simulink model "BACKUP"  (R2023b)
settings: Solver=VariableStepAuto  StartTime=0.0  StopTime=10.0  RelTol=1e-3
values from neighbouring files (symbols this model uses):
  C_PM = 1.758e-3    (= 0.001758)    [HVDCMMCInterconnectionParam.m]
  Carm = C_PM/Nb_PM    (= 4.88333333333e-05)    [HVDCMMCInterconnectionParam.m]
  Cfilter = 1/(Larm*wc2)    (= 4.78421193241e-05)    [HVDCMMCInterconnectionParam.m]
  Cg = 50e-9    (= 5e-08)    [HVDCMMCInterconnectionParam.m]
  Dd11 = Dd(1:nsw,1:nsw);        if(isempty(Dd11)) Dd11 = zeros(3,3); end    [DSS.m]    (also in DSS_test.m)
  Dd12 = Dd(1:nsw,nsw+1:end);    if(isempty(Dd12)) Dd12 = zeros(3,3); end    [DSS.m]    (also in DSS_test.m)
  Fnom = 50    [HVDCMMCInterconnectionParam.m]
  HRM = 2    [HVDCMMCInterconnectionParam.m]
  Ib_ac = (2/3)*Pnom/Vb_ac    [HVDCMMCInterconnectionParam.m]
  Ki_Ireg = 6    [HVDCMMCInterconnectionParam.m]
  Ki_Preg = 1.0    (= 1)    [HVDCMMCInterconnectionParam.m]
  Ki_Qreg = 1.0    (= 1)    [HVDCMMCInterconnectionParam.m]
  Ki_VDCreg = 100    [HVDCMMCInterconnectionParam.m]
  Kp_Ireg = 0.6    [HVDCMMCInterconnectionParam.m]
  Kp_Preg = 0.5/3    (= 0.166666666667)    [HVDCMMCInterconnectionParam.m]
  Kp_Qreg = 0.5/3    (= 0.166666666667)    [HVDCMMCInterconnectionParam.m]
  Kp_VDCreg = 4    [HVDCMMCInterconnectionParam.m]
  L_cable = 15e-3    (= 0.015)    [HVDCMMCInterconnectionParam.m]
  Larm = Larm_pu*(Zb_ac/(2*pi*Fnom))    [HVDCMMCInterconnectionParam.m]
  Lff = Larm_pu/2    (= 0.075)    [HVDCMMCInterconnectionParam.m]
  Limits_Ireg = [ 2.0  -2.0]    [HVDCMMCInterconnectionParam.m]
  Limits_Preg = [ 1.2, 0.8 ]    [HVDCMMCInterconnectionParam.m]
  Limits_Qreg = [ 0.25, -0.25 ]    [HVDCMMCInterconnectionParam.m]
  Limits_VDCreg = [ 2.0  -2.0]    [HVDCMMCInterconnectionParam.m]
  Lxfo = 0.12    [HVDCMMCInterconnectionParam.m]
  Nb_PM = 36    [HVDCMMCInterconnectionParam.m]
  Pnom = 1000e6    (= 1000000000)    [HVDCMMCInterconnectionParam.m]
  R_cable = 0.5    [HVDCMMCInterconnectionParam.m]
  R_startup = 400    [HVDCMMCInterconnectionParam.m]
  Rarm = Rarm_pu*Zb_ac    [HVDCMMCInterconnectionParam.m]
  Rff = Rarm_pu/2    (= 0.00075)    [HVDCMMCInterconnectionParam.m]
  Rfilter = 1/(Cfilter*w)*30    (= 1996.002)    [HVDCMMCInterconnectionParam.m]
  Rg = 100    [HVDCMMCInterconnectionParam.m]
  Rxfo = 0.003    [HVDCMMCInterconnectionParam.m]
  Ts = Ts_Control    (= 4e-05)    [HVDCMMCInterconnectionParam.m]
  Ts_Control = 40e-6    (= 4e-05)    [HVDCMMCInterconnectionParam.m]
  Ts_Power = 20e-6    (= 2e-05)    [HVDCMMCInterconnectionParam.m]
  Vb_ac = sqrt(2/3)*Vnom_sec    [HVDCMMCInterconnectionParam.m]
  Vc0_PM = 0    [HVDCMMCInterconnectionParam.m]
  Vnom_dc = 640e3    (= 640000)    [HVDCMMCInterconnectionParam.m]
  Vnom_prim = 400e3    (= 400000)    [HVDCMMCInterconnectionParam.m]
  Vnom_sec = 333e3    (= 333000)    [HVDCMMCInterconnectionParam.m]
  w = 2*pi*Fnom    (= 314.159265359)    [HVDCMMCInterconnectionParam.m]
  Zb_ac = Vb_ac/Ib_ac    [HVDCMMCInterconnectionParam.m]
undefined symbols (not defined in the file or in its folder): Ad1, Bd1, Cd1, DiscIntNeverNeededParam, gcbh, HrmOrd, Pcc, sps_AC, sps_ACDC, sps_rtmsupport, SYS, Ts_EMT
libraries: spsSeriesRLCBranchLib x22, simulink x20, spsCurrentMeasurementLib x13, spsControlledVoltageSourceLib x12, DQN_Lib x9, spsdq0toabcLib x3, powerlib_extras x3, spsGroundLib x3, spsBreakerLib x3, spsParallelRLCBranchLib x3, eeGeneralControl x2, dspspect3 x2
(part 1 of 5)
settings Model: Creator=rober  LastModifiedBy=rober

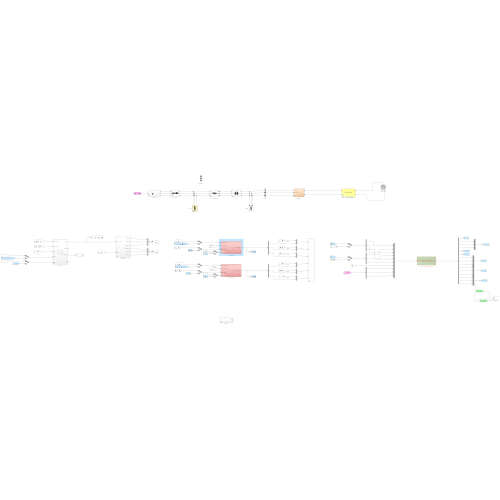
[thumbnail: Simulink's stored preview of the top-level diagram]
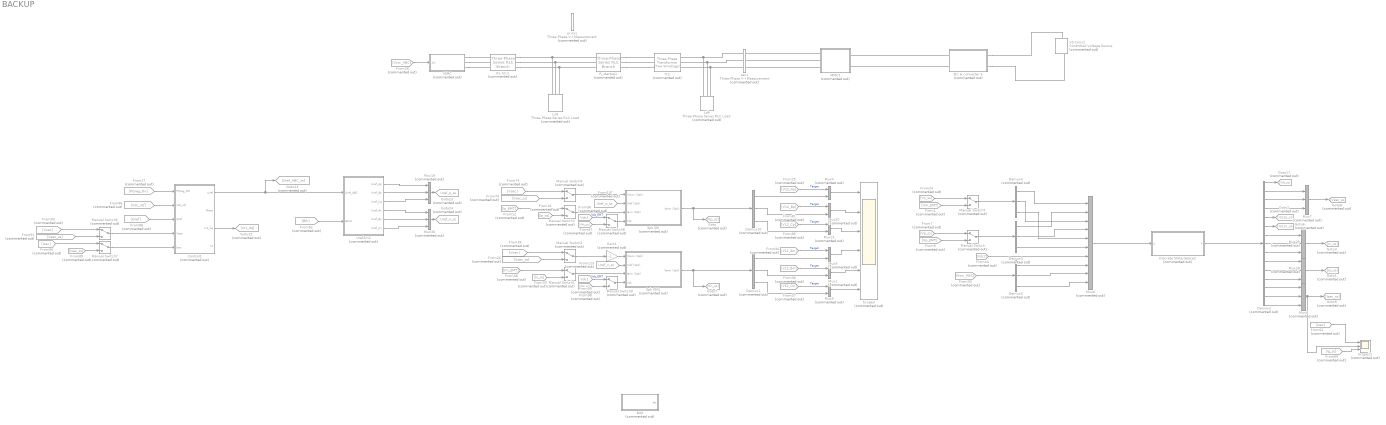
== system BACKUP ==
  3ph SM : Subsystem  Commented=on
  3ph SM1 : Subsystem  Commented=on
  BAK : Subsystem  Commented=on
  Control1 : Subsystem  Commented=on
  DC & converter 3 : Subsystem  Commented=on
      mask Display: disp('DC circuit')
  Demux{1,3..5,10} (5 alike) : Demux  Commented=on  Outputs=3
  Demux2 : Demux  Commented=on  Outputs=numel(sps_ACDC.outputs)
  Discrete State-Space2 : Subsystem  Commented=on  SystemSampleTime=Ts_Power  mask{A=sps_ACDC.A, B=sps_ACDC.B, C=sps_ACDC.C, D=sps_ACDC.D, InitVec=sps_ACDC.x0, dt=Ts_Power, DQSYM=off, N=HRM, Ws=w}
      mask prompts: InitVec "Initial condition:"; dt "Time step (s):"; N "Harmonic number:"; Ws "Angular frequency (1/rad):"
      mask init:
      | % I = eye(size(A,1));
      | % INVR = I/(I-A*dt/2);
      | % Ad1 = INVR*(I+A*dt/2);
      | % Bd1 = INVR*B*dt/2;
      | % Cd1 = C*Ad1;
      | % Dd11 = C*INVR*B*dt/2+D;
      | % Dd12 = C*INVR*B*dt/2;
      | 
      |     I = eye(size(A,1));
      |     INVR = I/(I-A*dt/2);
      |     Ad1 = INVR*(I+A*dt/2);
      |     Bd1 = INVR*B;
      |     Cd1 = C*INVR*dt;
      |     Dd1 = Cd1*B/2 + D;
      | 
      | DQSYM = get_param(gcb,'DQSYM');
      | 
      | comp = 0;
      | 
      | if(strcmp(DQSYM,'on'))
      | 
      | %Calculating the PNZ matrices
      | 
      |     a = -0.5+0.866i;
      |     a2 = -0.5-0.866i;
      |     Sas = [1,a,a2;1,a2,a;1,1,1]/3;
      | 
      |     arows = size(Ad1,1)/3; %signal size
      |     acols = size(Ad1,2)/3; %signal size
      | 
      |     brows = size(Bd1,1)/3; %signal size
      |     bcols = size(Bd1,2)/3; %signal size
      | 
      |     crows = size(Cd1,1)/3; %signal size
      |     ccols = size(Cd1,2)/3; %signal size
      | 
      |     d1rows = size(Dd1,1)/3; %signal size
      |     d1cols = size(Dd1,2)/3; %signal size
      | 
      |     %%%%%%%%%%%%%%%%%%%%%%% Check for inconsistencies  %%%%%%%%%%%%%%%%%%%%%%%
      | 
      |     szMatA = size(A,1);
      |     iL = eye(szMatA);
      |     szMatiL = size(iL,1);
      | 
      |     if(szMatiL ~= szMatA || size(A,1) ~= size(A,2) || size(iL,1) ~= size(iL,2))
      |         error('[Int_DQN_Mat/swFeedback] check matrix A size!');
      |     end
      | 
      |     if(arows ~= brows || acols ~= ccols || crows ~= d1rows || bcols ~= d1cols)
      |         error('[Int_DQN_Mat/Initialize] the sizes of the state-space matrices!');
      |     end
      | 
      |     %%%%%%%%%%%%%%%%%%%%%%%%%%%%%%%%%%%%%%%%%%%%%%%%%%%%%%%%%%%%%%%
      | 
      | 
      |     %%%%%%%%%%%%%%%%%%%%%%% A --> Bpnz %%%%%%%%%%%%%%%%%%%%%%%
      |     Adc = complex(zeros(3*arows,3*acols));
      | 
      |     for i = 1 : arows
      |         for j = 1 : acols
      |             Adc((1:3) + (i-1)*3,(1:3) + (j-1)*3) = Sas*Ad1((1:3) + (i-1)*3,(1:3) + (j-1)*3)/Sas;
      |             %Adc((1:3) + (i-1)*3,(1:3) + (j-1)*3) = diag(diag(real(Adc((1:3) + (i-1)*3,(1:3) + (j-1)*3))));
      |             %Adc((1:3) + (i-1)*3,(1:3) + (j-1)*3) = diag(diag((Adc((1:3) + (i-1)*3,(1:3) + (j-1)*3))));
      | 
      |         end
      |     end
      |     %%%%%%%%%%%%%%%%%%%%%%%%%%%%%%%%%%%%%%%%%%%%%%%%%%%%%%%%%%%%%%%
      | 
      |     %%%%%%%%%%%%%%%%%%%%%%% B --> Bpnz %%%%%%%%%%%%%%%%%%%%%%%
      | 
      |     Bdc = complex(zeros(3*brows,3*bcols));
      | 
      |     for i = 1 : brows
      |         for j = 1 : bcols
      |             Bdc((1:3) + (i-1)*3,(1:3) + (j-1)*3) = Sas*Bd1((1:3) + (i-1)*3,(1:3) + (j-1)*3)/Sas;
      |             %Bdc((1:3) + (i-1)*3,(1:3) + (j-1)*3) = diag(diag(real(Bdc((1:3) + (i-1)*3,(1:3) + (j-1)*3))));
      |             %Bdc((1:3) + (i-1)*3,(1:3) + (j-1)*3) = diag(diag((Bdc((1:3) + (i-1)*3,(1:3) + (j-1)*3))));
      | 
      |         end
      |     end
      |     %%%%%%%%%%%%%%%%%%%%%%%%%%%%%%%%%%%%%%%%%%%%%%%%%%%%%%%%%%%%%%%
      | 
      |     %%%%%%%%%%%%%%%%%%%%%%% C --> Cpnz %%%%%%%%%%%%%%%%%%%%%%%
      | 
      |     Cdc = complex(zeros(3*crows,3*ccols));
      | 
      |     for i = 1 : crows
      |         for j = 1 : ccols
      |             Cdc((1:3) + (i-1)*3,(1:3) + (j-1)*3) = Sas*Cd1((1:3) + (i-1)*3,(1:3) + (j-1)*3)/Sas;
      |             %Cdc((1:3) + (i-1)*3,(1:3) + (j-1)*3) = diag(diag(real(Cdc((1:3) + (i-1)*3,(1:3) + (j-1)*3))));
      |             %Cdc((1:3) + (i-1)*3,(1:3) + (j-1)*3) = diag(diag((Cdc((1:3) + (i-1)*3,(1:3) + (j-1)*3))));
      |         end
      |     end
      |     %%%%%%%%%%%%%%%%%%%%%%%%%%%%%%%%%%%%%%%%%%%%%%%%%%%%%%%%%%%%%%%
      | 
      |     
      |     %%%%%%%%%%%%%%%%%%%%%%% D1 --> Cpnz %%%%%%%%%%%%%%%%%%%%%%%
      | 
      |     Ddc = complex(zeros(3*d1rows,3*d1cols));
      | 
      |     for i = 1 : d1rows
      |         for j = 1 : d1cols
      |             Ddc((1:3) + (i-1)*3,(1:3) + (j-1)*3) = Sas*Dd1((1:3) + (i-1)*3,(1:3) + (j-1)*3)/Sas;
      |             %Ddc1((1:3) + (i-1)*3,(1:3) + (j-1)*3) = diag(diag(real(Ddc1((1:3) + (i-1)*3,(1:3) + (j-1)*3))));
      |             %Ddc((1:3) + (i-1)*3,(1:3) + (j-1)*3) = diag(diag((Ddc((1:3) + (i-1)*3,(1:3) + (j-1)*3))));
      |         end
      |     end
      |     %%%%%%%%%%%%%%%%%%%%%%%%%%%%%%%%%%%%%%%%%%%%%%%%%%%%%%%%%%%%%%%
      | 
      |     Adc(abs(Adc)<2*eps) = 0;
      |     Bdc(abs(Bdc)<2*eps) = 0;
      |     Cdc(abs(Cdc)<2*eps) = 0;
      |     Ddc(abs(Ddc)<2*eps) = 0;
      | 
      |     InitVec_c = complex(zeros(brows*3,N+1));
      | 
      | 
      |     if(~isempty(InitVec))
      |         if(mod(numel(InitVec),3)~=0) 
      |             warning('[SS_DQNc_Mat] InitVec with wrong size --> needs to be a multiple of 3!'); 
      | 
      |         else
      |             for k = 1 : numel(InitVec)/3
      |                 InitVec_c((k-1)*3+1:(k-1)*3+3,1) = Sas*InitVec((k-1)*3+1:(k-1)*3+3)*exp(+1i*Ws*dt);
      |             end
      |         end
      |     end
      | 
      |     InitVec = InitVec_c;
      | 
      | 
      |     Ad1 = Adc;
      |     Bd1 = Bdc;
      |     Cd1 = Cdc;
      |     Dd1 = Ddc;
      | 
      |     comp = -1i*Ws*dt;
      | 
      | end
      settings: MinAlgLoopOccurrences=on
      settings: LibrarySourceBlock=|
      | spsSynchronousMachineModel/Discrete robust/State Space Model/Discretize
      | BE or Tustin
      mask Callback DQSYM:
      | EMT = get_param(gcb,'DQSYM');
      | 
      | if(strcmp(EMT,'on'))
      |    set_param(gcb,'MaskVisibilities',{'on','on','on','on','on','on','on','on','on'});
      | else
      |    set_param(gcb,'MaskVisibilities',{'on','on','on','on','on','on','on','off','off'});
      | end
      mask Display: disp(['{\color{red}\bf\fontsize{12}x(t) = Ad*x(t-dt)+Bd*u(t)}',newline,'{\color{gray}\bf\fontsize{12}y(t) = Cd*x(t-dt)+Dd*u(t)}'], 'texmode','on');
  From1 : From  Commented=on  GotoTag=Vm_EMT
  From107 : From  Commented=on  GotoTag=Uref_p_ss  TagVisibility=global
  From113 : From  Commented=on  GotoTag=Uref_n_ss  TagVisibility=global
  From12 : From  Commented=on  GotoTag=Ip_EMT
  From16 : From  Commented=on  GotoTag=Ip_ss
  From24 : From  Commented=on  GotoTag=Vn_ss
  From25 : From  Commented=on  GotoTag=V12_Ap  TagVisibility=global
  From26 : From  Commented=on  GotoTag=Vsec_ss
  From27 : From  Commented=on  GotoTag=PQreg_On  TagVisibility=global
  From28 : From  Commented=on  GotoTag=Vsrc_ABC
  From30 : From  Commented=on  GotoTag=Vsrc_ABC
  From33 : From  Commented=on  GotoTag=In_ss
  From34 : From  Commented=on  GotoTag=V12_Am  TagVisibility=global
  From36 : From  Commented=on  GotoTag=V12_Bm  TagVisibility=global
  From37 : From  Commented=on  GotoTag=V12_Cm  TagVisibility=global
  From39 : From  Commented=on  GotoTag=Vsec  TagVisibility=global
  From44 : From  Commented=on  GotoTag=Vdc2  TagVisibility=global
  From48 : From  Commented=on  GotoTag=Im_EMT
  From62 : From  Commented=on  GotoTag=Isec  TagVisibility=global
  From69 : From  Commented=on  GotoTag=Ig_ss
  From7 : From  Commented=on  GotoTag=Vp_ss
  From73 : From  Commented=on  GotoTag=Vsec_ss
  From74 : From  Commented=on  GotoTag=Vsec  TagVisibility=global
  From81 : From  Commented=on  GotoTag=V12_Bp  TagVisibility=global
  From85 : From  Commented=on  GotoTag=V12_Cp  TagVisibility=global
  From86 : From  Commented=on  GotoTag=Vdc_ref  TagVisibility=global
  From87 : From  Commented=on  GotoTag=Vdc_ss
  From88 : From  Commented=on  GotoTag=Qref  TagVisibility=global
  From89 : From  Commented=on  GotoTag=Isec_ss
  From9 : From  Commented=on  GotoTag=Vp_EMT
  From90 : From  Commented=on  GotoTag=Isec  TagVisibility=global
  From91 : From  Commented=on  GotoTag=Vsec_ss
  From92 : From  Commented=on  GotoTag=Blk  TagVisibility=global
  From93 : From  Commented=on  GotoTag=Vsec  TagVisibility=global
  From96 : From  Commented=on  GotoTag=Vdc1  TagVisibility=global
  From98 : From  Commented=on  GotoTag=Vdc_ss
  From99 : From  Commented=on  GotoTag=Vdc1  TagVisibility=global
  Gain1 : Gain  Commented=on  Gain=-1
  Goto : Goto  Commented=on  GotoTag=Vp_ss
  Goto1 : Goto  Commented=on  GotoTag=Ip_ss
  Goto13 : Goto  Commented=on  GotoTag=Uref_ABC_ss
  Goto15 : Goto  Commented=on  GotoTag=m1_dq
  Goto17 : Goto  Commented=on  GotoTag=Vdc_ss
  Goto2 : Goto  Commented=on  GotoTag=Idc1p_ss
  Goto23 : Goto  Commented=on  GotoTag=Uref_p_ss  TagVisibility=global
  Goto24 : Goto  Commented=on  GotoTag=Uref_n_ss  TagVisibility=global
  Goto3 : Goto  Commented=on  GotoTag=In_ss
  Goto6 : Goto  Commented=on  GotoTag=Idc1n_ss
  Goto7 : Goto  Commented=on  GotoTag=Vn_ss
  Goto8 : Goto  Commented=on  GotoTag=Vsec_ss
  Goto9 : Goto  Commented=on  GotoTag=Isec_ss
  Ld3 : spsThreePhaseSeriesRLCLoadLib/Three-Phase Series RLC Load  Commented=on  LConnTagsString=A|B|C  Configuration=Y (grounded)  NominalVoltage=Vnom_prim  Vabc=[1e3 1e3 1e3]  Vabcp=[1e3 1e3 1e3]  NominalFrequency=Fnom  UnbalancedPower=off  ActivePower=P_Ld1  InductivePower=0  CapacitivePower=0  Pabc=[10e3 9e3 11e3]  QLabc=[100 90 110]  QCabc=[100 90 110]  Pabcp=[10e3 9e3 11e3]  QLabcp=[100 90 110]  QCabcp=[100 90 110]  Measurements=None  LoadType=constant Z
  Ld4 : spsThreePhaseSeriesRLCLoadLib/Three-Phase Series RLC Load  Commented=on  LConnTagsString=A|B|C  Configuration=Y (grounded)  NominalVoltage=Vnom_sec  Vabc=[1e3 1e3 1e3]  Vabcp=[1e3 1e3 1e3]  NominalFrequency=Fnom  UnbalancedPower=off  ActivePower=500e3  InductivePower=0  CapacitivePower=0  Pabc=[10e3 9e3 11e3]  QLabc=[100 90 110]  QCabc=[100 90 110]  Pabcp=[10e3 9e3 11e3]  QLabcp=[100 90 110]  QCabcp=[100 90 110]  Measurements=None  LoadType=constant Z
  MMC1 : Subsystem  Commented=on
  Manual Switch{,1..9} (10 alike) : ManualSwitch  Commented=on
  Mux{1,4..5,9,20..21} (6 alike) : Mux  Commented=on  Inputs=2
  Mux{7..8,19,28..30} (6 alike) : Mux  Commented=on  Inputs=3
  Mux6 : Mux  Commented=on  Inputs=numel(sps_ACDC.inputs)
  RL Src1 : spsThreePhaseSeriesRLCBranchLib/Three-Phase Series RLC Branch  Commented=on  LConnTagsString=A|B|C  RConnTagsString=A|B|C  BranchType=RL  Resistance=0.8929  Inductance=16.58e-3  Capacitance=1e-6  Measurements=None
  R_startup1 : spsThreePhaseSeriesRLCBranchLib/Three-Phase Series RLC Branch  Commented=on  LConnTagsString=A|B|C  RConnTagsString=A|B|C  BranchType=R  Resistance=R_startup/50  Inductance=Vnom_prim^2 / Pcc / (2*pi*Fnom)  Capacitance=1e-6  Measurements=None
  Scope11 : Scope  Commented=on  NumInputPorts=3
  Scope3 : Scope  Commented=on  NumInputPorts=6
  Tr2 : spsThreePhaseTransformerTwoWindingsLib/Three-Phase Transformer (Two Windings)  Commented=on  Winding1Connection=Yg  Winding2Connection=Yg  CoreType=Three single-phase transformers  SetSaturation=off  Hysteresis=off  DataFile='hysteresis'  SetInitialFlux=off  Measurements=None  UNITS=pu  NominalPower=[ Pnom , Fnom ]  Winding1="[ Vnom_prim , Rxfo/2,  Lxfo/2 ]"  Winding2="[ Vnom_sec , Rxfo/2,  Lxfo/2 ]"  Rm=1000  Lm=1000  L0=0.5  Saturation=[ 0,0 ; 0.0024,1.2 ; 1.0,1.52 ]  InitialFluxes=[ 0.8 , -0.8 , 0.7 ]  BreakLoop=off  DiscreteSolver=Trapezoidal iterative  DataType=off  TransfoNumber=1
  Uref2m2 : Subsystem  Commented=on
  VS Conv2 : spsControlledVoltageSourceLib/Controlled Voltage Source  Commented=on  Initialize=on  Source_Type=AC  Amplitude=0  Phase=0  Frequency=0  Measurements=None
  VSRC : Subsystem  Commented=on
  prim1 : spsThreePhaseVIMeasurementLib/Three-Phase V-I Measurement  Commented=on  VoltageMeasurement=phase-to-ground  SetLabelV=on  LabelV=Vprim  Vpu=off  VpuLL=off  CurrentMeasurement=yes  SetLabelI=on  LabelI=Iprim  Ipu=off  Pbase=100e6  Vbase=500e3  OutputType=Complex  PhasorSimulation=off  PSBequivalent=0
  sec1 : spsThreePhaseVIMeasurementLib/Three-Phase V-I Measurement  Commented=on  VoltageMeasurement=phase-to-ground  SetLabelV=on  LabelV=Vsec  Vpu=off  VpuLL=off  CurrentMeasurement=yes  SetLabelI=on  LabelI=Isec  Ipu=off  Pbase=100e6  Vbase=500e3  OutputType=Complex  PhasorSimulation=off  PSBequivalent=0
  wires:
  Gain1/1 -> 3ph SM1/1(Vconv (3ph))
  Demux10/3 -> Mux21/2
  Uref2m2/1(Uref_Ap) -> Mux19/1
  Demux4/1 -> Mux6/1
  Manual Switch9/1 -> 3ph SM1/4(Vdc)
  From25/1 -> Mux4/1  "Target"
  3ph SM1/1(Varm (3ph)) -> Goto7/1, Demux1/1
  Demux2/13 -> Mux8/1
  Mux30/1 -> Goto24/1
  Manual Switch/1 -> Demux3/1
  From16/1 -> Manual Switch3/2
  Demux5/1 -> Mux6/8
  From9/1 -> Manual Switch/2
  Uref2m2/2(Uref_Bp) -> Mux19/2
  Demux1/2 -> Mux1/2
  Demux2/6 -> Goto6/1
  From73/1 -> Manual Switch4/2
  From93/1 -> Manual Switch6/1
  From89/1 -> Manual Switch7/2
  From24/1 -> Manual Switch5/1
  Mux21/1 -> Scope3/3
  From107/1 -> 3ph SM/2(Vref (3ph))
  Uref2m2/4(Uref_An) -> Mux30/1
  Control1/3(m1_dq) -> Goto15/1
  From98/1 -> Manual Switch9/2
  Demux2/7 -> Mux29/1
  From37/1 -> Mux5/1  "Target"
  From87/1 -> Manual Switch8/2
  From96/1 -> Manual Switch8/1  "Vdc_EMT"
  Control1/1(Uref) -> Goto13/1, Uref2m2/1(Uref_ABC)
  Uref2m2/3(Uref_Cp) -> Mux19/3
  From90/1 -> Manual Switch7/1
  From92/1 -> Uref2m2/2(Block)
  Demux2/8 -> Mux29/2
  Manual Switch5/1 -> Demux4/1
  Mux1/1 -> Scope3/5
  From86/1 -> Control1/2(Vdc_ref)
  From88/1 -> Control1/3(Qref)
  Mux19/1 -> Goto23/1
  Manual Switch7/1 -> Control1/5(Isec)
  Manual Switch6/1 -> Control1/4(Vsec)
  Mux4/1 -> Scope3/1
  Uref2m2/5(Uref_Bn) -> Mux30/2
  From1/1 -> Manual Switch5/2
  From48/1 -> Manual Switch1/1
  From74/1 -> Manual Switch4/1
  Manual Switch3/1 -> 3ph SM/3(Iarm (3ph))
  Demux1/1 -> Mux9/2
  From113/1 -> 3ph SM1/2(Vref (3ph))
  Manual Switch1/1 -> 3ph SM1/3(Iarm (3ph))
  From33/1 -> Manual Switch1/2
  From39/1 -> Manual Switch2/1
  Demux5/2 -> Mux6/9
  From26/1 -> Manual Switch2/2
  Manual Switch2/1 -> Gain1/1
  Demux2/9 -> Mux29/3
  Demux1/3 -> Mux5/2
  Mux5/1 -> Scope3/6
  Demux2/5 -> Goto2/1
  From12/1 -> Manual Switch3/1
  Mux29/1 -> Goto3/1
  From44/1 -> Mux6/7
  From85/1 -> Mux21/1  "Target"
  Mux20/1 -> Scope3/2
  Demux10/1 -> Mux4/2
  From81/1 -> Mux20/1  "Target"
  Demux3/1 -> Mux6/2
  Discrete State-Space2/1(Y) -> Demux2/1
  Mux8/1 -> Goto9/1, Scope11/2
  From69/1 -> Scope11/3
  3ph SM/1(Varm (3ph)) -> Demux10/1, Goto/1
  From99/1 -> Manual Switch9/1  "Vdc_EMT"
  Demux2/1 -> Goto17/1
  Mux7/1 -> Goto8/1
  Demux2/3 -> Mux7/2
  Demux2/4 -> Mux7/3
  Demux2/11 -> Mux28/2
  From91/1 -> Manual Switch6/2
  Demux2/10 -> Mux28/1
  Demux2/2 -> Mux7/1
  From7/1 -> Manual Switch/1
  From30/1 -> Demux5/1
  Demux5/3 -> Mux6/10
  Manual Switch4/1 -> 3ph SM/1(Vconv (3ph))
  Demux4/2 -> Mux6/3
  Demux4/3 -> Mux6/5
  Manual Switch8/1 -> 3ph SM/4(Vdc)
  Demux2/15 -> Mux8/3
  From28/1 -> VSRC/1(In1)
  Mux6/1 -> Discrete State-Space2/1(U)
  Demux2/12 -> Mux28/3
  From27/1 -> Control1/1(PQreg_ON)
  Demux3/2 -> Mux6/4
  Demux2/14 -> Mux8/2
  From36/1 -> Mux1/1  "Target"
  Demux3/3 -> Mux6/6
  Mux28/1 -> Goto1/1
  Uref2m2/6(Uref_Cn) -> Mux30/3
  Mux9/1 -> Scope3/4
  From34/1 -> Mux9/1  "Target"
  Demux10/2 -> Mux20/2
  From62/1 -> Scope11/1
  connections:
  Ld3/LConn3 -- RL Src1/RConn3 -- R_startup1/LConn3
  Ld4/LConn2 -- Tr2/RConn2 -- sec1/RConn2
  Ld3/LConn2 -- RL Src1/RConn2 -- R_startup1/LConn2
  Ld3/LConn1 -- RL Src1/RConn1 -- R_startup1/LConn1
  Ld4/LConn3 -- Tr2/RConn3 -- sec1/RConn3
  Ld4/LConn1 -- Tr2/RConn1 -- sec1/RConn1
  DC & converter 3/RConn1 -- VS Conv2/RConn1
  VSRC/RConn2 -- RL Src1/LConn2
  DC & converter 3/LConn2 -- MMC1/RConn2
  DC & converter 3/RConn2 -- VS Conv2/LConn1
  VSRC/RConn3 -- RL Src1/LConn3
  MMC1/LConn1 -- sec1/LConn1
  MMC1/LConn2 -- sec1/LConn2
  DC & converter 3/LConn1 -- MMC1/RConn1
  R_startup1/RConn3 -- Tr2/LConn3
  VSRC/RConn1 -- RL Src1/LConn1
  R_startup1/RConn1 -- Tr2/LConn1
  R_startup1/RConn2 -- Tr2/LConn2
  MMC1/LConn3 -- sec1/LConn3

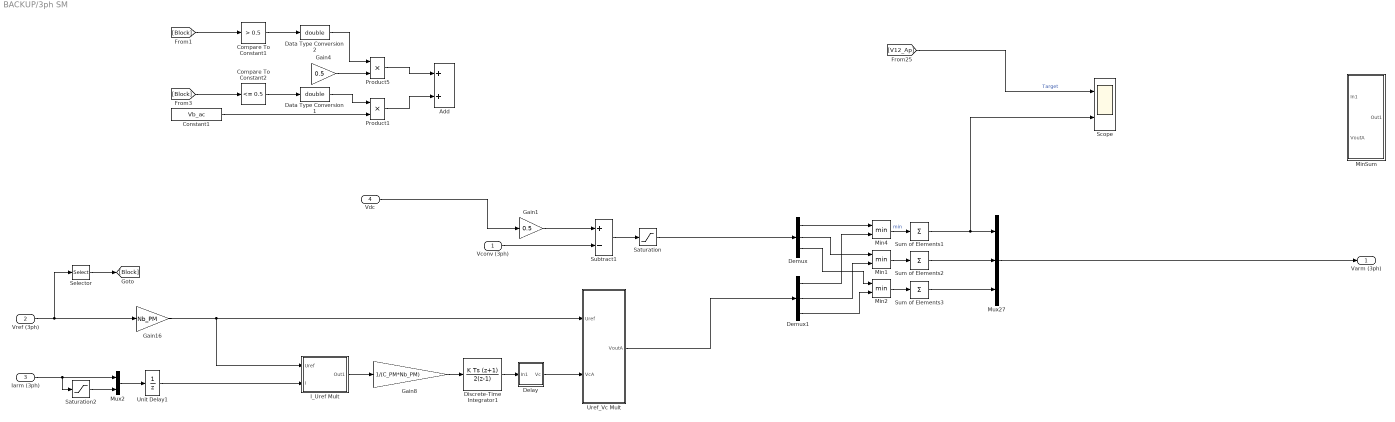
== system BACKUP/3ph SM ==
  Vconv (3ph) : Inport
  Vref (3ph) : Inport  Port=2
  Iarm (3ph) : Inport  Port=3
  Vdc : Inport  Port=4
  Add : Sum
  Compare To Constant1 : simulink/Logic and Bit Operations/Compare To Constant  relop=>  const=0.5  OutDataTypeStr=boolean
  Compare To Constant2 : simulink/Logic and Bit Operations/Compare To Constant  relop=<=  const=0.5  OutDataTypeStr=boolean
  Constant1 : Constant  Value=Vb_ac
  Data Type Conversion1 : DataTypeConversion  OutDataTypeStr=double  SaturateOnIntegerOverflow=off  RndMeth=Floor
  Data Type Conversion2 : DataTypeConversion  OutDataTypeStr=double  SaturateOnIntegerOverflow=off  RndMeth=Floor
  Delay : Subsystem
  Demux : Demux  Outputs=3
  Demux1 : Demux  Outputs=3
  Discrete-Time Integrator1 : DiscreteIntegrator  IntegratorMethod=Integration: Trapezoidal  gainval=1  SampleTime=Ts_Power  UpperSaturationLimit=5000  LowerSaturationLimit=500  ICPrevOutput=DiscIntNeverNeededParam  ICPrevScaledInput=DiscIntNeverNeededParam
  Gain1 : Gain  Gain=0.5
  Gain16 : Gain  Gain=Nb_PM
  Gain4 : Gain  Gain=0.5
  Gain8 : Gain  Gain=1/(C_PM*Nb_PM)
  I_Uref Mult : Subsystem
  Min1 : MinMax  Inputs=2
  Min2 : MinMax  Inputs=2
  Min4 : MinMax  Inputs=2
  MinSum : Subsystem
  Mux2 : Mux  Inputs=2
  Mux27 : Mux  Inputs=3
  Product1 : Product
  Product5 : Product
  Saturation : Saturate  UpperLimit=inf  LowerLimit=0
  Saturation2 : Saturate  UpperLimit=inf  LowerLimit=0
  Scope : Scope  NumInputPorts=2
  Selector : Selector  InputPortWidth=6  IndexOptions=Index vector (dialog)  Indices=2  OutputSizes=1
  Subtract1 : Sum  Inputs=+-
  Sum of Elements1 : Sum  Inputs=+
  Sum of Elements2 : Sum  Inputs=+
  Sum of Elements3 : Sum  Inputs=+
  Unit Delay1 : UnitDelay  SampleTime=Ts_Power  HasFrameUpgradeWarning=on
  Uref_Vc Mult : Subsystem
  Varm (3ph) : Outport
  wires:
  Subtract1/1 -> Saturation/1
  Vref (3ph)/1 -> Selector/1, Gain16/1
  Mux27/1 -> Varm (3ph)/1
  Gain8/1 -> Discrete-Time Integrator1/1
  Discrete-Time Integrator1/1 -> Delay/1(In1)
  Delay/1(Vc) -> Uref_Vc Mult/2(VcA)
  Gain16/1 -> I_Uref Mult/1(Uref), Uref_Vc Mult/1(Uref)
  Saturation2/1 -> Mux2/2
  Iarm (3ph)/1 -> Saturation2/1, Mux2/1
  Mux2/1 -> Unit Delay1/1
  Unit Delay1/1 -> I_Uref Mult/2(I)
  I_Uref Mult/1(Out1) -> Gain8/1
  Gain4/1 -> Product5/2
  [Block] -> Compare To Constant1/1
  Data Type Conversion2/1 -> Product5/1
  Compare To Constant1/1 -> Data Type Conversion2/1
  Vconv (3ph)/1 -> Subtract1/2
  Product5/1 -> Add/1
  [Block] -> Compare To Constant2/1
  Data Type Conversion1/1 -> Product1/1
  Compare To Constant2/1 -> Data Type Conversion1/1
  Constant1/1 -> Product1/2
  Product1/1 -> Add/2
  Vdc/1 -> Gain1/1
  Selector/1 -> [Block]
  Sum of Elements1/1 -> Scope/2, Mux27/1
  Demux1/1 -> Min4/2
  Demux1/3 -> Min2/2
  Demux1/2 -> Min1/2
  Saturation/1 -> Demux/1
  Demux/1 -> Min4/1
  Uref_Vc Mult/1(VoutA) -> Demux1/1
  Demux/2 -> Min1/1
  Sum of Elements3/1 -> Mux27/3
  Min1/1 -> Sum of Elements2/1
  Sum of Elements2/1 -> Mux27/2
  Demux/3 -> Min2/1
  Min4/1 -> Sum of Elements1/1  "min"
  Min2/1 -> Sum of Elements3/1
  [V12_Ap] -> Scope/1  "Target"
  Gain1/1 -> Subtract1/1

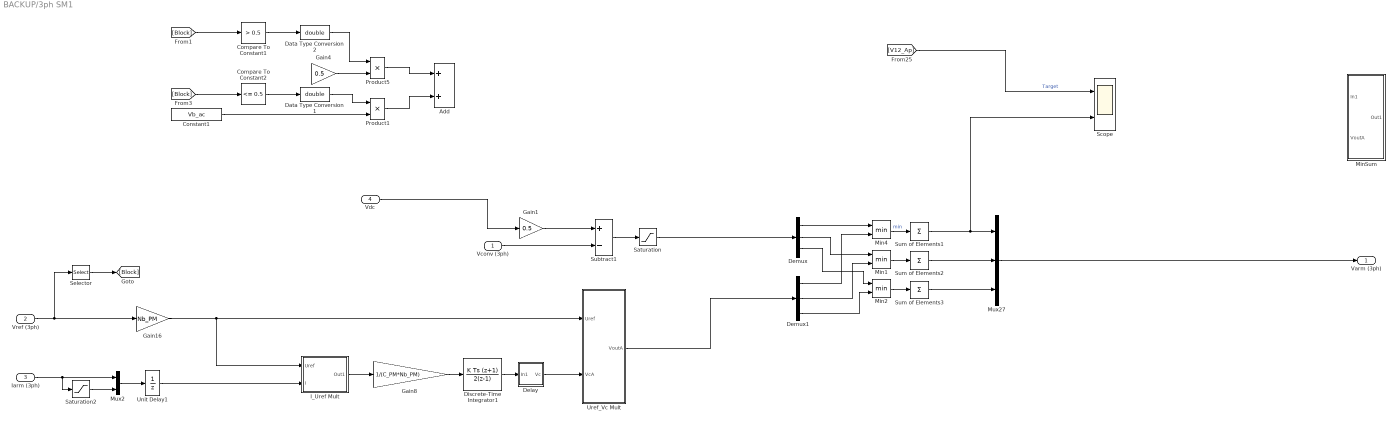
== system BACKUP/3ph SM1 ==
  Vconv (3ph) : Inport
  Vref (3ph) : Inport  Port=2
  Iarm (3ph) : Inport  Port=3
  Vdc : Inport  Port=4
  Add : Sum
  Compare To Constant1 : simulink/Logic and Bit Operations/Compare To Constant  relop=>  const=0.5  OutDataTypeStr=boolean
  Compare To Constant2 : simulink/Logic and Bit Operations/Compare To Constant  relop=<=  const=0.5  OutDataTypeStr=boolean
  Constant1 : Constant  Value=Vb_ac
  Data Type Conversion1 : DataTypeConversion  OutDataTypeStr=double  SaturateOnIntegerOverflow=off  RndMeth=Floor
  Data Type Conversion2 : DataTypeConversion  OutDataTypeStr=double  SaturateOnIntegerOverflow=off  RndMeth=Floor
  Delay : Subsystem
  Demux : Demux  Outputs=3
  Demux1 : Demux  Outputs=3
  Discrete-Time Integrator1 : DiscreteIntegrator  IntegratorMethod=Integration: Trapezoidal  gainval=1  SampleTime=Ts_Power  UpperSaturationLimit=5000  LowerSaturationLimit=500  ICPrevOutput=DiscIntNeverNeededParam  ICPrevScaledInput=DiscIntNeverNeededParam
  Gain1 : Gain  Gain=0.5
  Gain16 : Gain  Gain=Nb_PM
  Gain4 : Gain  Gain=0.5
  Gain8 : Gain  Gain=1/(C_PM*Nb_PM)
  I_Uref Mult : Subsystem
  Min1 : MinMax  Inputs=2
  Min2 : MinMax  Inputs=2
  Min4 : MinMax  Inputs=2
  MinSum : Subsystem
  Mux2 : Mux  Inputs=2
  Mux27 : Mux  Inputs=3
  Product1 : Product
  Product5 : Product
  Saturation : Saturate  UpperLimit=inf  LowerLimit=0
  Saturation2 : Saturate  UpperLimit=inf  LowerLimit=0
  Scope : Scope  NumInputPorts=2
  Selector : Selector  InputPortWidth=6  IndexOptions=Index vector (dialog)  Indices=2  OutputSizes=1
  Subtract1 : Sum  Inputs=+-
  Sum of Elements1 : Sum  Inputs=+
  Sum of Elements2 : Sum  Inputs=+
  Sum of Elements3 : Sum  Inputs=+
  Unit Delay1 : UnitDelay  SampleTime=Ts_Power  HasFrameUpgradeWarning=on
  Uref_Vc Mult : Subsystem
  Varm (3ph) : Outport
  wires:
  Subtract1/1 -> Saturation/1
  Vref (3ph)/1 -> Selector/1, Gain16/1
  Mux27/1 -> Varm (3ph)/1
  Gain8/1 -> Discrete-Time Integrator1/1
  Discrete-Time Integrator1/1 -> Delay/1(In1)
  Delay/1(Vc) -> Uref_Vc Mult/2(VcA)
  Gain16/1 -> I_Uref Mult/1(Uref), Uref_Vc Mult/1(Uref)
  Saturation2/1 -> Mux2/2
  Iarm (3ph)/1 -> Saturation2/1, Mux2/1
  Mux2/1 -> Unit Delay1/1
  Unit Delay1/1 -> I_Uref Mult/2(I)
  I_Uref Mult/1(Out1) -> Gain8/1
  Gain4/1 -> Product5/2
  [Block] -> Compare To Constant1/1
  Data Type Conversion2/1 -> Product5/1
  Compare To Constant1/1 -> Data Type Conversion2/1
  Vconv (3ph)/1 -> Subtract1/2
  Product5/1 -> Add/1
  [Block] -> Compare To Constant2/1
  Data Type Conversion1/1 -> Product1/1
  Compare To Constant2/1 -> Data Type Conversion1/1
  Constant1/1 -> Product1/2
  Product1/1 -> Add/2
  Vdc/1 -> Gain1/1
  Selector/1 -> [Block]
  Sum of Elements1/1 -> Scope/2, Mux27/1
  Demux1/1 -> Min4/2
  Demux1/3 -> Min2/2
  Demux1/2 -> Min1/2
  Saturation/1 -> Demux/1
  Demux/1 -> Min4/1
  Uref_Vc Mult/1(VoutA) -> Demux1/1
  Demux/2 -> Min1/1
  Sum of Elements3/1 -> Mux27/3
  Min1/1 -> Sum of Elements2/1
  Sum of Elements2/1 -> Mux27/2
  Demux/3 -> Min2/1
  Min4/1 -> Sum of Elements1/1  "min"
  Min2/1 -> Sum of Elements3/1
  [V12_Ap] -> Scope/1  "Target"
  Gain1/1 -> Subtract1/1
